simulink model "BPSK"  (R2023a)
settings: Solver=VariableStepAuto  StartTime=0.0  StopTime=10.0  RelTol=1e-3
values from neighbouring files (symbols this model uses):
  SNR_dB = 0:2:10    [hw3.m]
undefined symbols (not defined in the file or in its folder): k
libraries: commdigbbndpm3 x2, simulink x2, commchan3 x1, commrandsrc3 x1, commsink2 x1
settings Model: Creator=pds15  LastModifiedBy=pds15

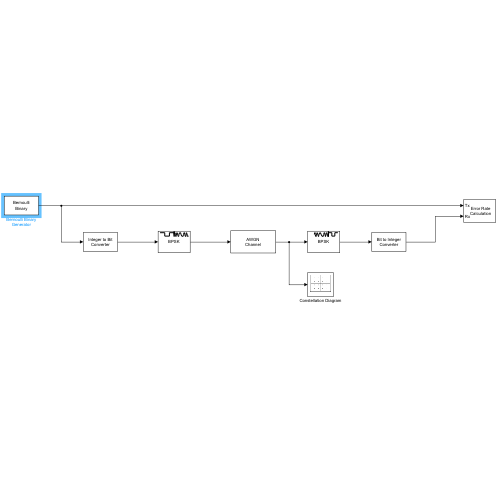
[thumbnail: Simulink's stored preview of the top-level diagram]
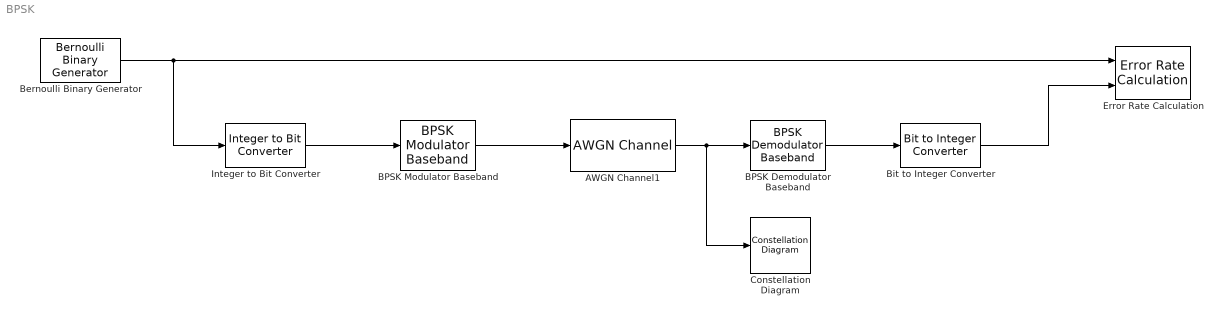
== system BPSK ==
  AWGN Channel1 : commchan3/AWGN Channel  LegacyMode=off  NoiseMethod="Signal to noise ratio  (SNR)"  noiseMode="Signal to noise ratio  (SNR)"  EbNo=10  EsNo=10  SNR=SNR_dB(k)  BitsPerSymbol=1  SignalPower=1  SamplesPerSymbol=1  SymbolPeriod=1  VarianceSource=Parameter  Variance=1  RandomStream=Global stream  Seed=67  SimulateUsing=Interpreted execution
  BPSK Demodulator Baseband : commdigbbndpm3/BPSK Demodulator Baseband  DecType=Hard decision  VarSource=Dialog  Variance=1  Ph=0  outDtype=Inherit via internal rule  derotateFactorWordLen=16  derotateFactorDataTypeStr=Inherit: Same word length as input  derotateFactorLastDataTypeStr=Inherit: Same word length as input
  BPSK Modulator Baseband : commdigbbndpm3/BPSK Modulator Baseband  Ph=0  outDtype=double  outWordLen=16  outUDDataType=sfix(16)  outFracLenMode=Best precision  outFracLen=15  outDataTypeStr=double  outLastDataTypeStr=double
  Bernoulli Binary Generator : commrandsrc3/Bernoulli Binary Generator  ProbabilityOfZero=0.5  SeedSource=Auto  Seed=0  SampleTime=0.00001  SamplesPerFrame=1000  OutputDataType=double  SimulateUsing=Interpreted execution
  Bit to Integer Converter : simulink/Logic and Bit Operations/Bit to Integer Converter  nbits=1  bitOrder=MSB first  signedOutputValues=Unsigned  outDtype=Inherit via internal rule  outDtypeSigned=Inherit via internal rule
  Constellation Diagram : ConstellationDiagram  WindowPosition=[447.000000,87.000000,600.000000,600.000000,]  ScopeFrameLocation=window
  Error Rate Calculation : commsink2/Error Rate Calculation  N=0  st_delay=0  cp_mode=Entire frame  subframe=[]  PMode=Workspace  WsName=ErrorVec  RsMode2=off  stop=off  numErr=100  maxBits=1e6
  Integer to Bit Converter : simulink/Logic and Bit Operations/Integer to Bit Converter  nbits=1  signedInputValues=Unsigned  bitOrder=MSB first  outDtype=Inherit via internal rule
  wires:
  BPSK Modulator Baseband/1 -> AWGN Channel1/1
  AWGN Channel1/1 -> Constellation Diagram/1, BPSK Demodulator Baseband/1
  Bernoulli Binary Generator/1 -> Error Rate Calculation/1, Integer to Bit Converter/1
  BPSK Demodulator Baseband/1 -> Bit to Integer Converter/1
  Bit to Integer Converter/1 -> Error Rate Calculation/2
  Integer to Bit Converter/1 -> BPSK Modulator Baseband/1
